simulink model "Model_samochodu"  (R2013a)
settings: Solver=ode113  StartTime=0.0  StopTime=1000  FixedStep=0.001  RelTol=1e-3
undefined symbols (not defined in the file): sigbuilder_block
settings Model: Creator=Damian  LastModifiedBy=Damian
settings SolverCC: ShapePreserveControl=EnableAll
settings DataIOCC: SignalLoggingSaveFormat=ModelDataLogs
settings OptimizationCC: BooleanDataType=off  InitFltsAndDblsToZero=on
settings HardwareCC: TargetHWDeviceType=32-bit Generic
settings GRTTargetCC: CombineOutputUpdateFcns=off  GRTInterface=on

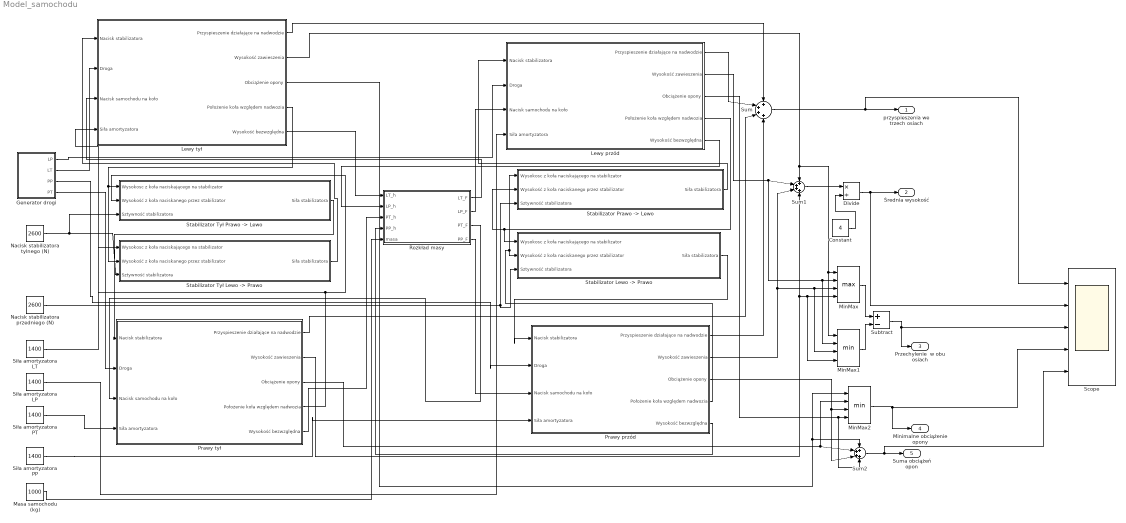
== system Model_samochodu ==
  Constant : Constant  Value=4
  Divide : Product  Inputs=*/
  Generator drogi : Subsystem
  Lewy przód : Subsystem
  Lewy tył : Subsystem
  Masa samochodu (kg) : Constant  Value=1000
  MinMax : MinMax  Function=max  Inputs=4
  MinMax1 : MinMax  Inputs=4
  MinMax2 : MinMax  Inputs=4
  Nacisk stabilizatora przedniego (N) : Constant  Value=2600
  Nacisk stabilizatora tylnego (N) : Constant  Value=2600
  Prawy przód : Subsystem
  Prawy tył : Subsystem
  Rozkład masy : Subsystem
  Scope : Scope  NumInputPorts=5
      settings: YMin=-5~-5~-5~-5~-5  YMax=5~5~5~5~5  SaveName=ScopeData6
  Siła amortyzatora LP : Constant  Value=1400
  Siła amortyzatora LT : Constant  Value=1400
  Siła amortyzatora PP : Constant  Value=1400
  Siła amortyzatora PT : Constant  Value=1400
  "Stabilizator Lewo -> Prawo" : Subsystem
  "Stabilizator Prawo -> Lewo" : Subsystem
  "Stabilizator Tył Lewo -> Prawo" : Subsystem
  "Stabilizator Tył Prawo -> Lewo" : Subsystem
  Subtract : Sum  Inputs=+-
  Sum : Sum  Inputs=++++
  Sum1 : Sum  Inputs=++++
  Sum2 : Sum  Inputs=++++
  przyspieszenia we trzech osiach : Outport
  "Średnia wysokość " : Outport  Port=2
  Przechylenie  w obu osiach : Outport  Port=3
  Minimalne obciążenie opony : Outport  Port=4
  "Suma obciążeń opon " : Outport  Port=5
  wires:
  Generator drogi/2(LT) -> Lewy tył/2(Droga)
  Generator drogi/1(LP) -> Lewy przód/2(Droga)
  Generator drogi/4(PT) -> Prawy tył/2(Droga)
  Generator drogi/3(PP) -> Prawy przód/2(Droga)
  Masa samochodu (kg)/1 -> Rozkład masy/5(masa)
  Rozkład masy/1(LT_F) -> Lewy tył/3(Nacisk samochodu na koło)
  Rozkład masy/2(LP_F) -> Lewy przód/3(Nacisk samochodu na koło)
  Rozkład masy/3(PT_F) -> Prawy tył/3(Nacisk samochodu na koło)
  Rozkład masy/4(PP_F) -> Prawy przód/3(Nacisk samochodu na koło)
  Lewy przód/4(Położenie koła względem nadwozia) -> "Stabilizator Prawo -> Lewo"/2(Wysokość z koła naciskanego przez stabilizator), "Stabilizator Lewo -> Prawo"/1(Wysokosc z koła naciskającego na stabilizator)
  Prawy przód/4(Położenie koła względem nadwozia) -> "Stabilizator Prawo -> Lewo"/1(Wysokosc z koła naciskającego na stabilizator), "Stabilizator Lewo -> Prawo"/2(Wysokość z koła naciskanego przez stabilizator)
  "Stabilizator Lewo -> Prawo"/1(Siła stabilizatora) -> Prawy przód/1(Nacisk stabilizatora)
  "Stabilizator Prawo -> Lewo"/1(Siła stabilizatora) -> Lewy przód/1(Nacisk stabilizatora)
  Lewy tył/4(Położenie koła względem nadwozia) -> "Stabilizator Tył Lewo -> Prawo"/2(Wysokość z koła naciskanego przez stabilizator), "Stabilizator Tył Prawo -> Lewo"/1(Wysokosc z koła naciskającego na stabilizator)
  Prawy tył/4(Położenie koła względem nadwozia) -> "Stabilizator Tył Prawo -> Lewo"/2(Wysokość z koła naciskanego przez stabilizator), "Stabilizator Tył Lewo -> Prawo"/1(Wysokosc z koła naciskającego na stabilizator)
  "Stabilizator Tył Prawo -> Lewo"/1(Siła stabilizatora) -> Prawy tył/1(Nacisk stabilizatora)
  "Stabilizator Tył Lewo -> Prawo"/1(Siła stabilizatora) -> Lewy tył/1(Nacisk stabilizatora)
  Nacisk stabilizatora tylnego (N)/1 -> "Stabilizator Tył Lewo -> Prawo"/3(Sztywność stabilizatora), "Stabilizator Tył Prawo -> Lewo"/3(Sztywność stabilizatora)
  Nacisk stabilizatora przedniego (N)/1 -> "Stabilizator Lewo -> Prawo"/3(Sztywność stabilizatora), "Stabilizator Prawo -> Lewo"/3(Sztywność stabilizatora)
  Siła amortyzatora LT/1 -> Lewy tył/4(Siła amortyzatora)
  Siła amortyzatora PT/1 -> Prawy tył/4(Siła amortyzatora)
  Siła amortyzatora LP/1 -> Lewy przód/4(Siła amortyzatora)
  Siła amortyzatora PP/1 -> Prawy przód/4(Siła amortyzatora)
  Lewy tył/5("Wysokość bezwzględna ") -> Rozkład masy/1(LT_h)
  Lewy przód/5("Wysokość bezwzględna ") -> Rozkład masy/2(LP_h)
  Prawy tył/5("Wysokość bezwzględna ") -> Rozkład masy/3(PT_h)
  Prawy przód/5("Wysokość bezwzględna ") -> Rozkład masy/4(PP_h)
  Lewy tył/1(Przyspieszenie działające na nadwodzie) -> Sum/1
  Lewy przód/1(Przyspieszenie działające na nadwodzie) -> Sum/2
  Prawy tył/1(Przyspieszenie działające na nadwodzie) -> Sum/3
  Prawy przód/1(Przyspieszenie działające na nadwodzie) -> Sum/4
  Sum/1 -> Scope/1, przyspieszenia we trzech osiach/1
  Lewy tył/2(Wysokość zawieszenia) -> MinMax/1, MinMax1/1, Sum1/1
  Lewy przód/2(Wysokość zawieszenia) -> MinMax1/2, MinMax/2, Sum1/2
  Prawy przód/2(Wysokość zawieszenia) -> MinMax1/3, MinMax/3, Sum1/3
  Prawy tył/2(Wysokość zawieszenia) -> MinMax1/4, MinMax/4, Sum1/4
  Sum1/1 -> Divide/1
  Constant/1 -> Divide/2
  Divide/1 -> "Średnia wysokość "/1, Scope/2
  MinMax/1 -> Subtract/1
  MinMax1/1 -> Subtract/2
  Subtract/1 -> Scope/3, Przechylenie  w obu osiach/1
  Lewy tył/3(Obciążenie opony) -> MinMax2/1, Sum2/1
  Prawy tył/3(Obciążenie opony) -> MinMax2/2, Sum2/2
  Prawy przód/3(Obciążenie opony) -> Sum2/3, MinMax2/3
  Lewy przód/3(Obciążenie opony) -> Sum2/4, MinMax2/4
  MinMax2/1 -> Scope/4, Minimalne obciążenie opony/1
  Sum2/1 -> Scope/5, "Suma obciążeń opon "/1

== system Model_samochodu/Generator drogi ==
  Signal Builder : Subsystem  Tag=STV Subsys  LoadFcn=sigbuilder_block('load');  StartFcn=sigbuilder_block('start');  StopFcn=sigbuilder_block('stop');  ClipboardFcn=sigbuilder_block('clipboard');  mask(Sigbuilder block){}
      mask help: Create and generate interchangeable groups of signals whose waveforms are piecewise linear.
      mask init:
      | if ~strcmp(get_param(bdroot(gcbh),'SimulationStatus'),'stopped') tuvar = sigbuilder_block('maskInit'); end
      settings: CopyFcn=sigbuilder_block('copy');  DeleteFcn=sigbuilder_block('delete');  ModelCloseFcn=sigbuilder_block('modelClose');  PreSaveFcn=sigbuilder_block('preSave');  PauseFcn=sigbuilder_block('pause')  ContinueFcn=sigbuilder_block('continue')  NameChangeFcn=sigbuilder_block('namechange');  OpenFcn=sigbuilder_block('open',[108 122.25 550.5 390 ]);  CloseFcn=sigbuilder_block('close');
      mask Display: plot(0,0,100,100,[10,10,40,40,10],[80,20,20,80,80],[40,10],[50,50], [40,27,10],[65,72,56],[40,25,25,10],[28,28,43,43]);
  Signal Builder1 : Subsystem  Tag=STV Subsys  LoadFcn=sigbuilder_block('load');  StartFcn=sigbuilder_block('start');  StopFcn=sigbuilder_block('stop');  ClipboardFcn=sigbuilder_block('clipboard');  mask(Sigbuilder block){}
      mask help: Simulink:masks:SigbuilderBlock_MD
      mask init:
      | if ~strcmp(get_param(bdroot(gcbh),'SimulationStatus'),'stopped') tuvar = sigbuilder_block('maskInit'); end
      settings: CopyFcn=sigbuilder_block('copy');  DeleteFcn=sigbuilder_block('delete');  ModelCloseFcn=sigbuilder_block('modelClose');  PreSaveFcn=sigbuilder_block('preSave');  PauseFcn=sigbuilder_block('pause');  ContinueFcn=sigbuilder_block('continue');  NameChangeFcn=sigbuilder_block('namechange');  OpenFcn=sigbuilder_block('open',[0 30 1258.5 678.75 ]);  CloseFcn=sigbuilder_block('close');
      mask Display: plot(0, 0, 100, 100,[2, 2, 32, 32, 2], [68, 8, 8, 68, 68],[32, 2], [38, 38], [32, 19, 2],[53, 60, 44], [32, 17, 17, 2],[16, 16, 31, 31]);txt = getActiveGroup(gcbh);text(2, 100, txt,'verticalAlignment', 'top');
  Transport Delay1 : TransportDelay  DelayTime=0.27  BufferSize=102400
  Transport Delay2 : TransportDelay  DelayTime=0.27  BufferSize=102400
  LP : Outport
  LT : Outport  Port=2
  PP : Outport  Port=3
  PT : Outport  Port=4
  wires:
  Signal Builder1/1(Lewe koło) -> Transport Delay1/1, LP/1
  Transport Delay1/1 -> LT/1
  Transport Delay2/1 -> PT/1
  Signal Builder1/2(Prawe koło) -> Transport Delay2/1, PP/1

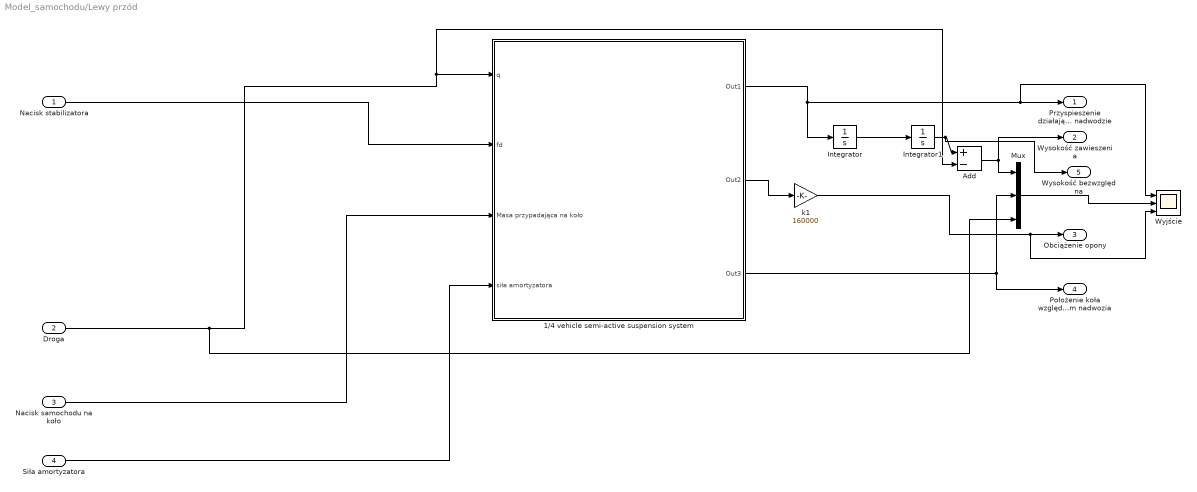
== system Model_samochodu/Lewy przód ==
  Nacisk stabilizatora : Inport
  Droga : Inport  Port=2
  Nacisk samochodu na koło : Inport  Port=3
  Siła amortyzatora : Inport  Port=4
  1/4 vehicle semi-active suspension system : Subsystem
      mask Display: image(imread('Semi_acitve model2DOF.jpg'));
  Add : Sum  Inputs=+-
  Integrator : Integrator
  Integrator1 : Integrator
  Mux : Mux  Inputs=3
  Wyjście : Scope  NumInputPorts=3
      settings: YMin=-40~-0.4~-20000  YMax=40~0.4~20000  SaveName=ScopeData3
  k1 : Gain  Gain=160000  SaturateOnIntegerOverflow=on  OutDataTypeStr=Inherit: Same as input  ParamDataTypeStr=Inherit: Same as input
  Przyspieszenie działające na nadwodzie : Outport
  Wysokość zawieszenia : Outport  Port=2
  Obciążenie opony : Outport  Port=3
  Położenie koła względem nadwozia : Outport  Port=4
  "Wysokość bezwzględna " : Outport  Port=5
  wires:
  1/4 vehicle semi-active suspension system/1(Out1) -> Integrator/1, Wyjście/1, Przyspieszenie działające na nadwodzie/1
  1/4 vehicle semi-active suspension system/3(Out3) -> Mux/2, Położenie koła względem nadwozia/1
  1/4 vehicle semi-active suspension system/2(Out2) -> k1/1
  k1/1 -> Wyjście/3, Obciążenie opony/1
  Integrator/1 -> Integrator1/1
  Mux/1 -> Wyjście/2
  Droga/1 -> Mux/3, 1/4 vehicle semi-active suspension system/1(q), Add/2
  Nacisk samochodu na koło/1 -> 1/4 vehicle semi-active suspension system/3(Masa przypadająca na koło)
  Nacisk stabilizatora/1 -> 1/4 vehicle semi-active suspension system/2(fd)
  Integrator1/1 -> "Wysokość bezwzględna "/1, Add/1
  Add/1 -> Mux/1, Wysokość zawieszenia/1
  Siła amortyzatora/1 -> 1/4 vehicle semi-active suspension system/4(siła amortyzatora)

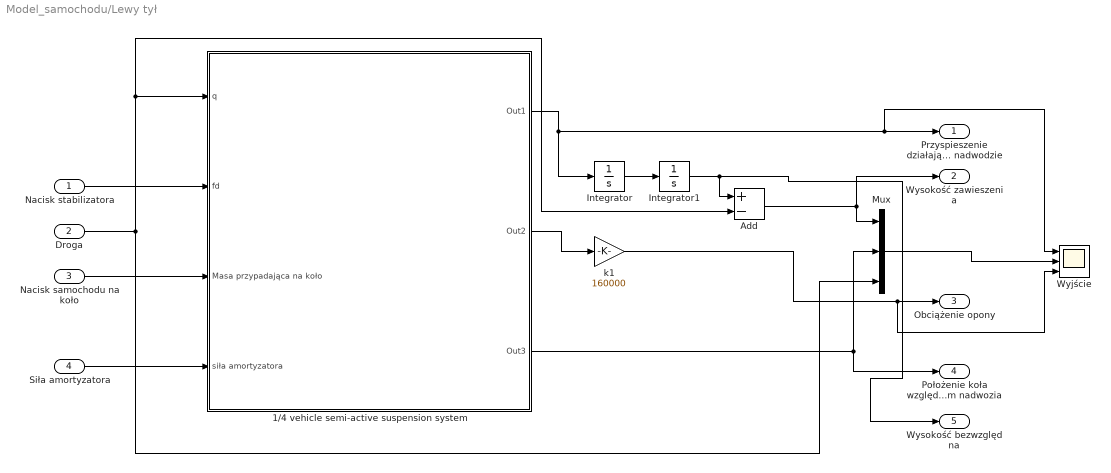
== system Model_samochodu/Lewy tył ==
  Nacisk stabilizatora : Inport
  Droga : Inport  Port=2
  Nacisk samochodu na koło : Inport  Port=3
  Siła amortyzatora : Inport  Port=4
  1/4 vehicle semi-active suspension system : Subsystem
      mask Display: image(imread('Semi_acitve model2DOF.jpg'));
  Add : Sum  Inputs=+-
  Integrator : Integrator
  Integrator1 : Integrator
  Mux : Mux  Inputs=3
  Wyjście : Scope  NumInputPorts=3
      settings: YMin=-40~-0.4~-20000  YMax=40~0.4~20000
  k1 : Gain  Gain=160000  SaturateOnIntegerOverflow=on  OutDataTypeStr=Inherit: Same as input  ParamDataTypeStr=Inherit: Same as input
  Przyspieszenie działające na nadwodzie : Outport
  Wysokość zawieszenia : Outport  Port=2
  Obciążenie opony : Outport  Port=3
  Położenie koła względem nadwozia : Outport  Port=4
  "Wysokość bezwzględna " : Outport  Port=5
  wires:
  1/4 vehicle semi-active suspension system/1(Out1) -> Wyjście/1, Przyspieszenie działające na nadwodzie/1, Integrator/1
  1/4 vehicle semi-active suspension system/3(Out3) -> Mux/2, Położenie koła względem nadwozia/1
  1/4 vehicle semi-active suspension system/2(Out2) -> k1/1
  k1/1 -> Wyjście/3, Obciążenie opony/1
  Integrator/1 -> Integrator1/1
  Mux/1 -> Wyjście/2
  Droga/1 -> 1/4 vehicle semi-active suspension system/1(q), Add/2, Mux/3
  Nacisk samochodu na koło/1 -> 1/4 vehicle semi-active suspension system/3(Masa przypadająca na koło)
  Nacisk stabilizatora/1 -> 1/4 vehicle semi-active suspension system/2(fd)
  Integrator1/1 -> "Wysokość bezwzględna "/1, Add/1
  Add/1 -> Mux/1, Wysokość zawieszenia/1
  Siła amortyzatora/1 -> 1/4 vehicle semi-active suspension system/4(siła amortyzatora)

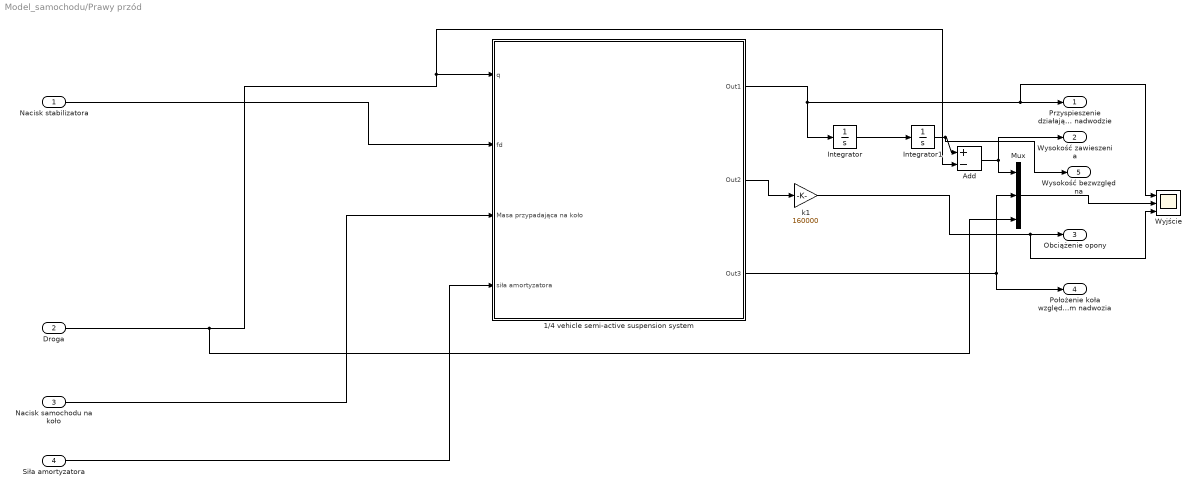
== system Model_samochodu/Prawy przód ==
  Nacisk stabilizatora : Inport
  Droga : Inport  Port=2
  Nacisk samochodu na koło : Inport  Port=3
  Siła amortyzatora : Inport  Port=4
  1/4 vehicle semi-active suspension system : Subsystem
      mask Display: image(imread('Semi_acitve model2DOF.jpg'));
  Add : Sum  Inputs=+-
  Integrator : Integrator
  Integrator1 : Integrator
  Mux : Mux  Inputs=3
  Wyjście : Scope  NumInputPorts=3
      settings: YMin=-40~-0.4~-20000  YMax=40~0.4~20000  SaveName=ScopeData5
  k1 : Gain  Gain=160000  SaturateOnIntegerOverflow=on  OutDataTypeStr=Inherit: Same as input  ParamDataTypeStr=Inherit: Same as input
  Przyspieszenie działające na nadwodzie : Outport
  Wysokość zawieszenia : Outport  Port=2
  Obciążenie opony : Outport  Port=3
  Położenie koła względem nadwozia : Outport  Port=4
  "Wysokość bezwzględna " : Outport  Port=5
  wires:
  1/4 vehicle semi-active suspension system/1(Out1) -> Integrator/1, Wyjście/1, Przyspieszenie działające na nadwodzie/1
  1/4 vehicle semi-active suspension system/3(Out3) -> Mux/2, Położenie koła względem nadwozia/1
  1/4 vehicle semi-active suspension system/2(Out2) -> k1/1
  k1/1 -> Wyjście/3, Obciążenie opony/1
  Integrator/1 -> Integrator1/1
  Mux/1 -> Wyjście/2
  Droga/1 -> Mux/3, 1/4 vehicle semi-active suspension system/1(q), Add/2
  Nacisk samochodu na koło/1 -> 1/4 vehicle semi-active suspension system/3(Masa przypadająca na koło)
  Nacisk stabilizatora/1 -> 1/4 vehicle semi-active suspension system/2(fd)
  Integrator1/1 -> "Wysokość bezwzględna "/1, Add/1
  Add/1 -> Mux/1, Wysokość zawieszenia/1
  Siła amortyzatora/1 -> 1/4 vehicle semi-active suspension system/4(siła amortyzatora)

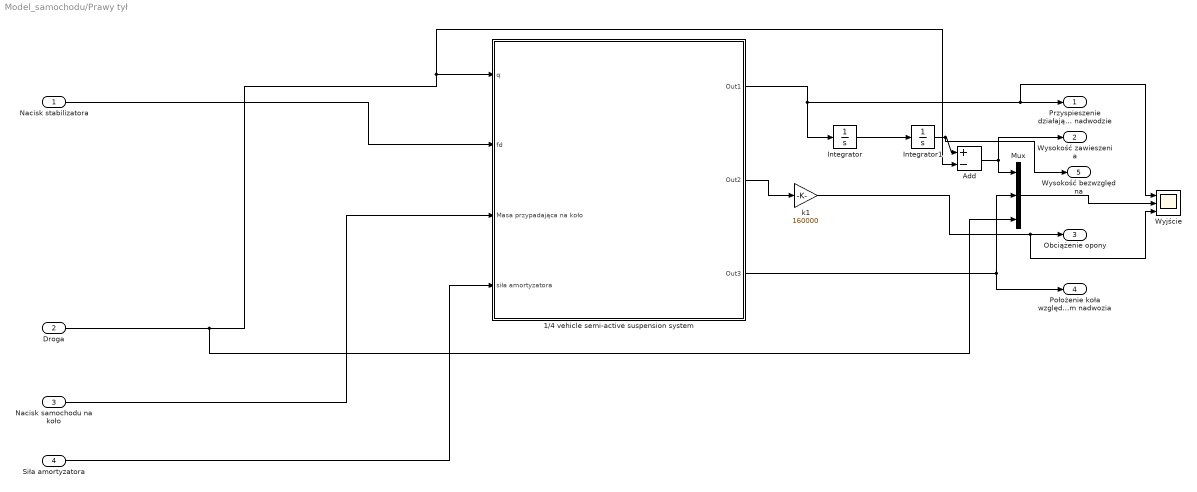
== system Model_samochodu/Prawy tył ==
  Nacisk stabilizatora : Inport
  Droga : Inport  Port=2
  Nacisk samochodu na koło : Inport  Port=3
  Siła amortyzatora : Inport  Port=4
  1/4 vehicle semi-active suspension system : Subsystem
      mask Display: image(imread('Semi_acitve model2DOF.jpg'));
  Add : Sum  Inputs=+-
  Integrator : Integrator
  Integrator1 : Integrator
  Mux : Mux  Inputs=3
  Wyjście : Scope  NumInputPorts=3
      settings: YMin=-40~-0.4~-20000  YMax=40~0.4~20000  SaveName=ScopeData2
  k1 : Gain  Gain=160000  SaturateOnIntegerOverflow=on  OutDataTypeStr=Inherit: Same as input  ParamDataTypeStr=Inherit: Same as input
  Przyspieszenie działające na nadwodzie : Outport
  Wysokość zawieszenia : Outport  Port=2
  Obciążenie opony : Outport  Port=3
  Położenie koła względem nadwozia : Outport  Port=4
  "Wysokość bezwzględna " : Outport  Port=5
  wires:
  1/4 vehicle semi-active suspension system/1(Out1) -> Integrator/1, Wyjście/1, Przyspieszenie działające na nadwodzie/1
  1/4 vehicle semi-active suspension system/3(Out3) -> Mux/2, Położenie koła względem nadwozia/1
  1/4 vehicle semi-active suspension system/2(Out2) -> k1/1
  k1/1 -> Wyjście/3, Obciążenie opony/1
  Integrator/1 -> Integrator1/1
  Mux/1 -> Wyjście/2
  Droga/1 -> Mux/3, 1/4 vehicle semi-active suspension system/1(q), Add/2
  Nacisk samochodu na koło/1 -> 1/4 vehicle semi-active suspension system/3(Masa przypadająca na koło)
  Nacisk stabilizatora/1 -> 1/4 vehicle semi-active suspension system/2(fd)
  Integrator1/1 -> "Wysokość bezwzględna "/1, Add/1
  Add/1 -> Mux/1, Wysokość zawieszenia/1
  Siła amortyzatora/1 -> 1/4 vehicle semi-active suspension system/4(siła amortyzatora)

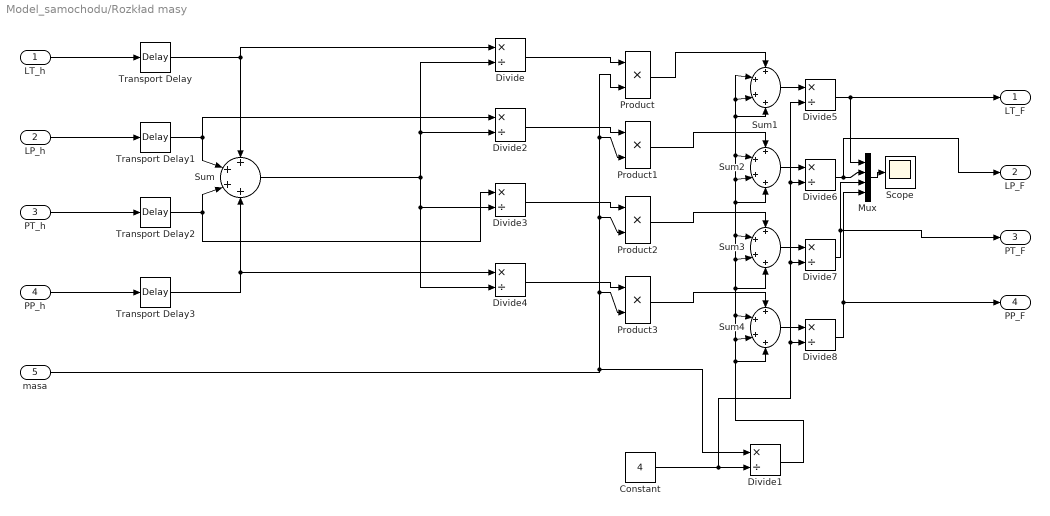
== system Model_samochodu/Rozkład masy ==
  LT_h : Inport
  LP_h : Inport  Port=2
  PT_h : Inport  Port=3
  PP_h : Inport  Port=4
  masa : Inport  Port=5
  Constant : Constant  Value=4
  Divide{,1..8} (9 alike) : Product  Inputs=*/
  Mux : Mux
  Product{,1..3} (4 alike) : Product
  Scope : Scope
      settings: TimeRange=1000  YMin=170  YMax=330
  Sum{,1..4} (5 alike) : Sum  Inputs=++++
  Transport Delay{,1..3} (4 alike) : TransportDelay  DelayTime=0.001  InitialOutput=1
  LT_F : Outport
  LP_F : Outport  Port=2
  PT_F : Outport  Port=3
  PP_F : Outport  Port=4
  wires:
  Sum/1 -> Divide4/2, Divide3/2, Divide2/2, Divide/2
  Divide/1 -> Product/1
  Divide2/1 -> Product1/1
  Divide3/1 -> Product2/1
  Divide4/1 -> Product3/1
  masa/1 -> Divide1/1, Product3/2, Product2/2, Product1/2, Product/2
  Mux/1 -> Scope/1
  Constant/1 -> Divide5/2, Divide6/2, Divide7/2, Divide8/2, Divide1/2
  Transport Delay/1 -> Sum/1, Divide/1
  Transport Delay1/1 -> Divide2/1, Sum/2
  Transport Delay2/1 -> Sum/3, Divide3/1
  Transport Delay3/1 -> Divide4/1, Sum/4
  LT_h/1 -> Transport Delay/1
  LP_h/1 -> Transport Delay1/1
  PT_h/1 -> Transport Delay2/1
  PP_h/1 -> Transport Delay3/1
  Product/1 -> Sum1/1
  Product1/1 -> Sum2/1
  Divide1/1 -> Sum4/4, Sum4/2, Sum3/4, Sum3/2, Sum2/4, Sum2/2, Sum1/4, Sum1/3, Sum1/2, Sum2/3, Sum3/3, Sum4/3
  Product2/1 -> Sum3/1
  Product3/1 -> Sum4/1
  Sum1/1 -> Divide5/1
  Sum2/1 -> Divide6/1
  Sum3/1 -> Divide7/1
  Sum4/1 -> Divide8/1
  Divide5/1 -> LT_F/1, Mux/1
  Divide8/1 -> PP_F/1, Mux/4
  Divide6/1 -> LP_F/1, Mux/2
  Divide7/1 -> PT_F/1, Mux/3

== system Model_samochodu/Stabilizator Lewo -> Prawo ==
  Wysokosc z koła naciskającego na stabilizator : Inport
  Wysokość z koła naciskanego przez stabilizator : Inport  Port=2
  Sztywność stabilizatora : Inport  Port=3
  Divide : Product  Inputs=**
  Gain : Gain  Gain=-1
  Subtract : Sum  Inputs=+-
  Siła stabilizatora : Outport
  wires:
  Wysokosc z koła naciskającego na stabilizator/1 -> Subtract/1
  Wysokość z koła naciskanego przez stabilizator/1 -> Subtract/2
  Subtract/1 -> Divide/1
  Sztywność stabilizatora/1 -> Divide/2
  Divide/1 -> Gain/1
  Gain/1 -> Siła stabilizatora/1

== system Model_samochodu/Stabilizator Prawo -> Lewo ==
  Wysokosc z koła naciskającego na stabilizator : Inport
  Wysokość z koła naciskanego przez stabilizator : Inport  Port=2
  Sztywność stabilizatora : Inport  Port=3
  Divide : Product  Inputs=**
  Gain : Gain  Gain=-1
  Subtract : Sum  Inputs=+-
  Siła stabilizatora : Outport
  wires:
  Wysokosc z koła naciskającego na stabilizator/1 -> Subtract/1
  Wysokość z koła naciskanego przez stabilizator/1 -> Subtract/2
  Subtract/1 -> Divide/1
  Sztywność stabilizatora/1 -> Divide/2
  Divide/1 -> Gain/1
  Gain/1 -> Siła stabilizatora/1

== system Model_samochodu/Stabilizator Tył Lewo -> Prawo ==
  Wysokosc z koła naciskającego na stabilizator : Inport
  Wysokość z koła naciskanego przez stabilizator : Inport  Port=2
  Sztywność stabilizatora : Inport  Port=3
  Divide : Product  Inputs=**
  Gain : Gain  Gain=-1
  Subtract : Sum  Inputs=+-
  Siła stabilizatora : Outport
  wires:
  Wysokosc z koła naciskającego na stabilizator/1 -> Subtract/1
  Wysokość z koła naciskanego przez stabilizator/1 -> Subtract/2
  Subtract/1 -> Divide/1
  Sztywność stabilizatora/1 -> Divide/2
  Divide/1 -> Gain/1
  Gain/1 -> Siła stabilizatora/1

== system Model_samochodu/Stabilizator Tył Prawo -> Lewo ==
  Wysokosc z koła naciskającego na stabilizator : Inport
  Wysokość z koła naciskanego przez stabilizator : Inport  Port=2
  Sztywność stabilizatora : Inport  Port=3
  Divide : Product  Inputs=**
  Gain : Gain  Gain=-1
  Subtract : Sum  Inputs=+-
  Siła stabilizatora : Outport
  wires:
  Wysokosc z koła naciskającego na stabilizator/1 -> Subtract/1
  Wysokość z koła naciskanego przez stabilizator/1 -> Subtract/2
  Subtract/1 -> Divide/1
  Sztywność stabilizatora/1 -> Divide/2
  Divide/1 -> Gain/1
  Gain/1 -> Siła stabilizatora/1

== system Model_samochodu/Generator drogi/Signal Builder ==
  Demux : Demux  Tag=STV Demux  Outputs=2
  FromWs : FromWorkspace  Tag=STV FromWs  VariableName=tuvar  SampleTime=0
      SigBuilderData=|
      | common.afterFinalStr = 'Extrapolate'
      | common.sampleTime = 0
      | dataSet.timeRange = [0 100]
      | dataSet.name = 'Arkusz1'
      | sbobj.Name = 'Signal Builder'
      | sbobj.Groups.Name = 'Arkusz1'
      | sbobj.Groups.Signals(1).Name = 'Imported_Signal 1'
      | sbobj.Groups.Signals(1).XData = [0 44.5 45 48 48 100]
      | sbobj.Groups.Signals(1).YData = [0 0 0.1 0.1 -0.001 0]
      | sbobj.Groups.Signals(2).Name = 'Imported_Signal 2'
      | sbobj.Groups.Signals(2).XData = [0 10 15 20 30 31 32 33 34 35 36 37 38 39 50 51 52 53 54 55 56 57 58 59 60 70 75 80 85 90 95 100]
      | sbobj.Groups.Signals(2).YData = [0 0.1 0.1 0 0.01 0.014 0.02 0.032 0.06 0.072 0.078 0.084 0.09 0.1 0.1 0.096 0.09 0.082 0.07 0.038 0.016 0.01 0.01 0.016 0.006 -0.1 -0.05 -0.05 0.02 0.03 0.02 0]
      | sbobj.Groups.TimeRange = [0 100]
  Imported_Signal 1 : Outport
  Imported_Signal 2 : Outport  Tag=STV Outport  Port=2
  wires:
  FromWs/1 -> Demux/1
  Demux/1 -> Imported_Signal 1/1
  Demux/2 -> Imported_Signal 2/1

== system Model_samochodu/Generator drogi/Signal Builder1 ==
  Demux : Demux  Tag=STV Demux  Outputs=2
  FromWs : FromWorkspace  Tag=STV FromWs  VariableName=tuvar  SampleTime=0
      SigBuilderData=|
      | common.afterFinalStr = 'Extrapolate'
      | common.sampleTime = 0
      | dataSet.timeRange = [0 1000]
      | dataSet.name = 'Group 1'
      | sbobj.Groups.Name = 'Group 1'
      | sbobj.Groups.Signals(1).Name = 'Lewe koło'
      | sbobj.Groups.Signals(1).XData = [0 20 20.5 21 22 40 40 41.5 42 60 60 61.5 61.5 75 75.5 76 76 77 77 78 78.5 79 79.5 80 80 81 81.5 82 82.5 83 83.5 84 84.5 85 85.5 86.5 87 88 89.5 90.5 91 91.5 92 93 93.5 94.5 95 95.5 96.5 97 97.5 98 110 110 111 111 112 112 113 113 114 114 115 115 130 131 133 135.5 137.5 138.5 140 160 161 164 167 170 172 190 190.5 191 191 192 192.5 193 206 207 208 208.5 209.5 210 211 212 213 227 228 229 230 230.5 231 231.5 232 232.5 233 233 233.5 235.5 236 237.5 238.5 239 240 241 247.5 248.5 249.5 250 251 252 252.5 253 269.5 271 273 275 277 278 280.5 283 285.5 288.5 291 294.5 297 300 303 308 312 313.5 315 317 318 319.5 321 328 331.5 334.5 338 344 344 358.5 359.5 361.5 363 364 366 367.5 369.5 371.5 374 377 379 382 384 385 400.5 400.5 403.5 403.5 415 415 417.5 417.5 432 432 435 436.5 439 440 442 446 449 480 481 483 484.5 487 489 491 493 495.5 498 500 501.5 504 505.5 506.5 508.5 509 510 524 564 571 628 660.5 660.5 664 664 668 668 671.5 671.5 676 676 679 679 682.5 682.5 686 686 689.5 689.5 692.5 692.5 697 697 701 701 706 706 711 711 715.5 715.5 720.5 720.5 751 753 756.5 760 763 767 771 774.5 778 782 787 791 796 799 800.3 800.3 800.5 800.5 800.75 800.75 801.05 801.05 801.2 801.2 801.35 801.35 801.5 801.5 801.6 801.6 801.75 801.75 801.95 801.95 802.2 802.2 802.4 802.4 802.7 802.7 802.95 802.95 803.2 803.2 803.5 803.5 803.7 803.7 803.85 803.85 804 804 804.2 804.2 804.4 804.4 804.65 804.65 804.85 804.85 805.1 805.1 805.36 805.36 805.58 805.58 805.72 805.72 805.92 805.92 806.06 806.06 806.22 806.22 806.38 806.38 806.56 806.56 806.78 806.78 806.94 806.94 807.08 807.08 807.24 807.24 807.44 807.44 807.6 807.6 807.78 807.78 807.98 807.98 810 814.5 815.8 820 825 829 834 841 843.2 846.5 851.5 856 862 867.8 867.8 872.8 872.8 877.2 879.6 887.4 893 899 904.6 910.4 917 923.4 930.4 936.2 942.6 948 954.8 959.4 965 971.6 977 984.6 989.6 994.2 1000]
      | sbobj.Groups.Signals(1).YData = [0.001 0.001 0.101 0.101 0.001 0.001 -0.1 -0.1 0 0 0.101 0.101 ... (368 elements, 1x368)]
      | sbobj.Groups.Signals(2).Name = 'Prawe koło'
      | sbobj.Groups.Signals(2).XData = [0 19.5 20 20.5 21 39.5 40 41 41.5 59.5 60 61 61.5 74.5 75 75.5 76.5 77.5 78.5 79.5 80.5 82 83 84 85 85 86 86.5 87.5 88.5 89.5 90 90.5 91.5 92.5 93.5 93.5 94.5 109.5 109.5 110.5 110.5 111 111 112 112 113.5 113.5 114.5 114.5 129.5 130.5 132.5 135 136.5 138.5 139.5 159.5 160.5 163.5 166.5 169.5 171 189.5 190 190.5 191 191.5 192 193 193.5 226.5 226.5 227.5 227.5 229.5 229.5 230.5 230.5 231 231 240 240 241.5 241.5 246.5 250 252 264.5 266.5 266.5 274 278.5 288.5 295.5 311.5 324 342.5 342.5 358 358 359 359 359.5 359.5 360.5 360.5 361.5 361.5 362 362 363 363 364 364 365 365 366 366 367.5 367.5 368 368 368.5 368.5 369.5 369.5 370.5 370.5 372 372 373 373 375 375 408.5 408.5 411 411 423 423 432 432 435 438 440.5 444 446.5 449 452.5 479.5 481 482.5 485.5 487.5 489.5 491 494.5 497 499.5 502 505.5 507 508.5 509.5 519.5 519.5 525 525 529.5 529.5 533 533 538 538 542.5 542.5 545.5 545.5 549.5 549.5 554.5 554.5 559 559 564 564 568.5 568.5 574.5 574.5 579.5 579.5 584 584 589.5 589.5 596 596 601 601 609 609 613.5 613.5 617.5 617.5 621.5 621.5 626 626 659.5 663.5 667.5 671.5 675.5 680 684.5 689.5 695 699.5 705 710 715 720 748 752.5 757 762 762 766 766 769 773 777 780.5 786.5 791.5 796.5 800 800.18 800.18 800.32 800.32 800.42 800.42 800.52 800.52 800.66 800.66 800.82 800.82 800.92 800.92 801.02 801.02 801.12 801.12 801.24 801.24 801.34 801.34 801.44 801.44 801.58 801.58 801.76 801.76 801.84 801.84 801.96 801.96 802.04 802.04 802.18 802.18 802.34 802.34 802.48 802.48 802.64 802.64 802.84 803.06 803.24 803.24 803.41 803.41 803.58 804 804 805.15 805.15 805.27 805.27 805.85 805.85 806.03 806.03 806.3 807 807 807.52 807.74 807.74 808.02 808.02 808.28 811.5 816.5 821 826 830.5 834 839.5 845 850 855 859 864.5 864.5 870 870 874.5 876.5 879.5 880.8 882.6 884.6 888.4 891.8 894 898.4 900.8 902.8 906.2 911 915 923.5 923.5 931 931 935.5 935.5 939 939 941 941 944 946.5 949.5 950.5 953.5 957 960 961.5 964 967 970 976 981 988 994 1000]
      | sbobj.Groups.Signals(2).YData = [-0.001 -0.001 0.099 0.099 -0.001 -0.001 -0.101 -0.1 -0.002 -0.001 -0.1 -0.099 ... (364 elements, 1x364)]
      | sbobj.Groups.TimeRange = [0 1000]
  Lewe koło : Outport  Tag=STV Outport
  Prawe koło : Outport  Tag=STV Outport  Port=2
  wires:
  Demux/1 -> Lewe koło/1
  FromWs/1 -> Demux/1
  Demux/2 -> Prawe koło/1

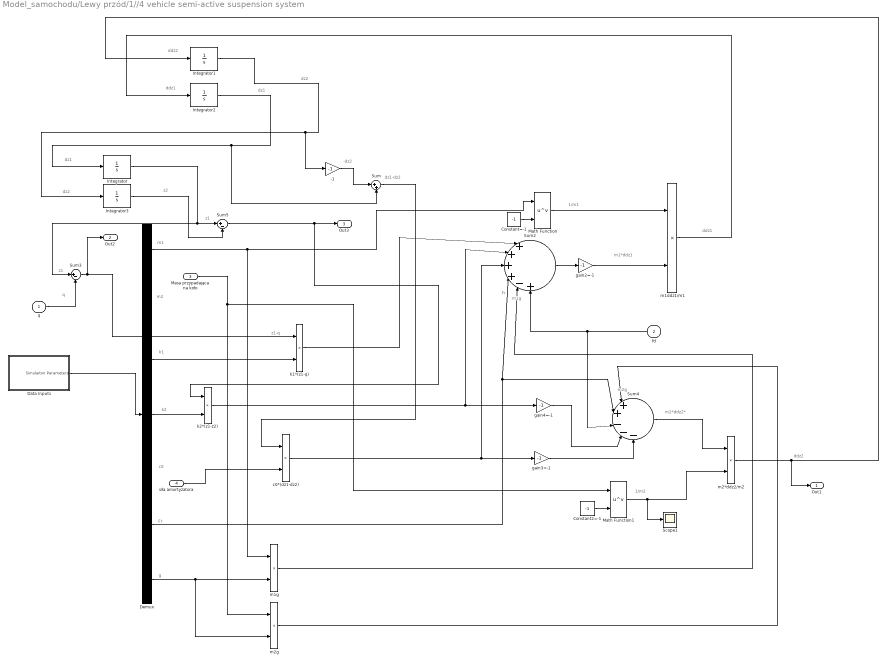
== system Model_samochodu/Lewy przód/1//4 vehicle semi-active suspension system ==
  note: m1
  note: k1
  note: m2
  note: k2
  note: c0
  note: z1
  note: dz1
  note: Fr
  note: g
  note: dz2
  note: -dz2
  note: dz1-dz2
  note: dz1
  note: dz2
  note: ddz2
  note: q
  note: z1
  note: z1-q
  note: Fr
  note: m1g
  note: m1*ddz1
  note: 1/m1
  note: ddz1
  note: m2g
  note: m2*ddz2*
  note: 1/m2
  note: ddz2
  note: z2
  note: ddz1
  q : Inport
  fd : Inport  Port=2
  Masa przypadająca na koło : Inport  Port=3
  siła amortyzatora : Inport  Port=4
  -1 : Gain  Gain=-1  SaturateOnIntegerOverflow=on  OutDataTypeStr=Inherit: Same as input  ParamDataTypeStr=Inherit: Same as input
  Constant2=-1 : Constant  Value=-1
  Constant=-1 : Constant  Value=-1
  Data Inputs : Subsystem
  Demux : Demux  Outputs=7
  Integrator{,1..3} (4 alike) : Integrator
  Math Function : Math  Operator=pow  SaturateOnIntegerOverflow=on
  Math Function1 : Math  Operator=pow  SaturateOnIntegerOverflow=on
  Scope1 : Scope
      settings: SaveName=ScopeData4
  Sum : Sum  Inputs=|++  SaturateOnIntegerOverflow=on  InputSameDT=on  OutDataTypeStr=Inherit: Same as first input
  Sum2 : Sum  Inputs=|++++-+  SaturateOnIntegerOverflow=on  InputSameDT=on  OutDataTypeStr=Inherit: Same as first input
  Sum3 : Sum  Inputs=|+-  SaturateOnIntegerOverflow=on  InputSameDT=on  OutDataTypeStr=Inherit: Same as first input
  Sum4 : Sum  Inputs=|++---  SaturateOnIntegerOverflow=on  InputSameDT=on  OutDataTypeStr=Inherit: Same as first input
  Sum5 : Sum  Inputs=|+-  SaturateOnIntegerOverflow=on  InputSameDT=on  OutDataTypeStr=Inherit: Same as first input
  c0*(dz1-dz2) : Product  SaturateOnIntegerOverflow=on  RndMeth=Zero  InputSameDT=on  OutDataTypeStr=Inherit: Same as first input
  gain2=-1 : Gain  Gain=-1  SaturateOnIntegerOverflow=on  OutDataTypeStr=Inherit: Same as input  ParamDataTypeStr=Inherit: Same as input
  gain3=-1 : Gain  Gain=-1  SaturateOnIntegerOverflow=on  OutDataTypeStr=Inherit: Same as input  ParamDataTypeStr=Inherit: Same as input
  gain4=-1 : Gain  Gain=-1  SaturateOnIntegerOverflow=on  OutDataTypeStr=Inherit: Same as input  ParamDataTypeStr=Inherit: Same as input
  k1*(z1-q) : Product  SaturateOnIntegerOverflow=on  RndMeth=Zero  InputSameDT=on  OutDataTypeStr=Inherit: Same as first input
  k2*(z1-z2) : Product  SaturateOnIntegerOverflow=on  RndMeth=Zero  InputSameDT=on  OutDataTypeStr=Inherit: Same as first input
  m1ddz1/m1 : Product  SaturateOnIntegerOverflow=on  RndMeth=Zero  InputSameDT=on  OutDataTypeStr=Inherit: Same as first input
  m1g : Product  SaturateOnIntegerOverflow=on  RndMeth=Zero  InputSameDT=on  OutDataTypeStr=Inherit: Same as first input
  m2*ddz2/m2 : Product  SaturateOnIntegerOverflow=on  RndMeth=Zero  InputSameDT=on  OutDataTypeStr=Inherit: Same as first input
  m2g : Product  SaturateOnIntegerOverflow=on  RndMeth=Zero  InputSameDT=on  OutDataTypeStr=Inherit: Same as first input
  Out1 : Outport
  Out2 : Outport  Port=2
  Out3 : Outport  Port=3
  wires:
  Data Inputs/1("Simulaiton Parameters ") -> Demux/1
  Demux/1 -> m1g/1, Math Function/1
  Integrator2/1 -> Sum/2, Integrator/1
  Integrator/1 -> Sum5/1, Sum3/1
  siła amortyzatora/1 -> c0*(dz1-dz2)/2
  -1/1 -> Sum/1
  Sum/1 -> c0*(dz1-dz2)/1
  Integrator1/1 -> -1/1, Integrator3/1
  Demux/4 -> k2*(z1-z2)/2
  Demux/3 -> k1*(z1-q)/2
  Sum3/1 -> k1*(z1-q)/1, Out2/1
  Sum2/1 -> gain2=-1/1
  gain2=-1/1 -> m1ddz1/m1/2
  k1*(z1-q)/1 -> Sum2/1
  k2*(z1-z2)/1 -> Sum2/2, gain4=-1/1
  c0*(dz1-dz2)/1 -> Sum2/3, gain3=-1/1
  fd/1 -> Sum2/6, Sum4/3
  Constant=-1/1 -> Math Function/2
  Math Function/1 -> m1ddz1/m1/1
  m1ddz1/m1/1 -> Integrator2/1
  Demux/6 -> Sum2/4, Sum4/2
  gain3=-1/1 -> Sum4/5
  gain4=-1/1 -> Sum4/4
  Sum4/1 -> m2*ddz2/m2/1
  Demux/7 -> m1g/2, m2g/2
  Masa przypadająca na koło/1 -> m2g/1, Math Function1/1
  m1g/1 -> Sum2/5
  m2g/1 -> Sum4/1
  Constant2=-1/1 -> Math Function1/2
  Math Function1/1 -> m2*ddz2/m2/2, Scope1/1
  m2*ddz2/m2/1 -> Integrator1/1, Out1/1
  Integrator3/1 -> Sum5/2
  Sum5/1 -> k2*(z1-z2)/1, Out3/1
  q/1 -> Sum3/2

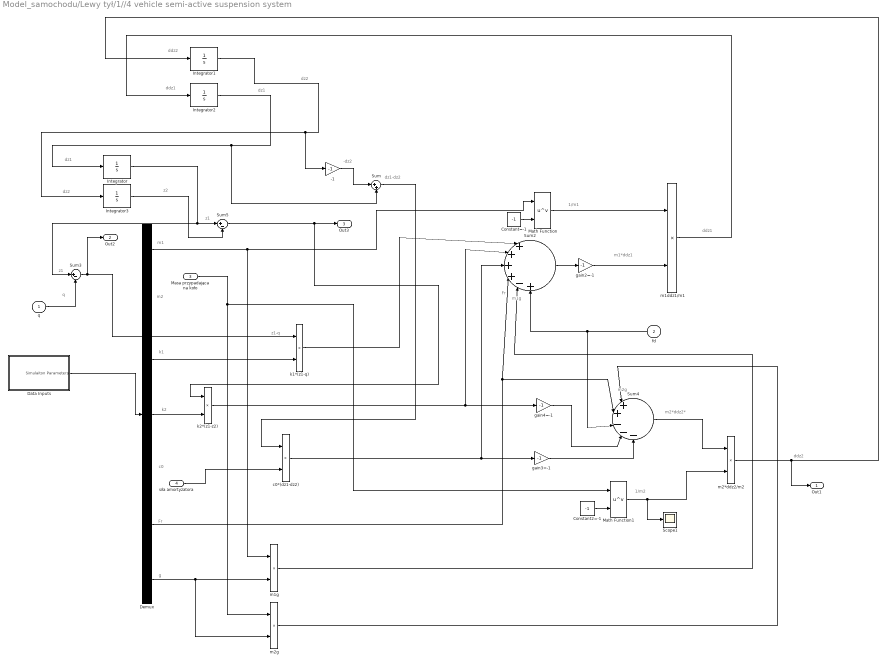
== system Model_samochodu/Lewy tył/1//4 vehicle semi-active suspension system ==
  note: m1
  note: k1
  note: m2
  note: k2
  note: c0
  note: z1
  note: dz1
  note: Fr
  note: g
  note: dz2
  note: -dz2
  note: dz1-dz2
  note: dz1
  note: dz2
  note: ddz2
  note: q
  note: z1
  note: z1-q
  note: Fr
  note: m1g
  note: m1*ddz1
  note: 1/m1
  note: ddz1
  note: m2g
  note: m2*ddz2*
  note: 1/m2
  note: ddz2
  note: z2
  note: ddz1
  q : Inport
  fd : Inport  Port=2
  Masa przypadająca na koło : Inport  Port=3
  siła amortyzatora : Inport  Port=4
  -1 : Gain  Gain=-1  SaturateOnIntegerOverflow=on  OutDataTypeStr=Inherit: Same as input  ParamDataTypeStr=Inherit: Same as input
  Constant2=-1 : Constant  Value=-1
  Constant=-1 : Constant  Value=-1
  Data Inputs : Subsystem
  Demux : Demux  Outputs=7
  Integrator{,1..3} (4 alike) : Integrator
  Math Function : Math  Operator=pow  SaturateOnIntegerOverflow=on
  Math Function1 : Math  Operator=pow  SaturateOnIntegerOverflow=on
  Scope1 : Scope
      settings: SaveName=ScopeData4
  Sum : Sum  Inputs=|++  SaturateOnIntegerOverflow=on  InputSameDT=on  OutDataTypeStr=Inherit: Same as first input
  Sum2 : Sum  Inputs=|++++-+  SaturateOnIntegerOverflow=on  InputSameDT=on  OutDataTypeStr=Inherit: Same as first input
  Sum3 : Sum  Inputs=|+-  SaturateOnIntegerOverflow=on  InputSameDT=on  OutDataTypeStr=Inherit: Same as first input
  Sum4 : Sum  Inputs=|++---  SaturateOnIntegerOverflow=on  InputSameDT=on  OutDataTypeStr=Inherit: Same as first input
  Sum5 : Sum  Inputs=|+-  SaturateOnIntegerOverflow=on  InputSameDT=on  OutDataTypeStr=Inherit: Same as first input
  c0*(dz1-dz2) : Product  SaturateOnIntegerOverflow=on  RndMeth=Zero  InputSameDT=on  OutDataTypeStr=Inherit: Same as first input
  gain2=-1 : Gain  Gain=-1  SaturateOnIntegerOverflow=on  OutDataTypeStr=Inherit: Same as input  ParamDataTypeStr=Inherit: Same as input
  gain3=-1 : Gain  Gain=-1  SaturateOnIntegerOverflow=on  OutDataTypeStr=Inherit: Same as input  ParamDataTypeStr=Inherit: Same as input
  gain4=-1 : Gain  Gain=-1  SaturateOnIntegerOverflow=on  OutDataTypeStr=Inherit: Same as input  ParamDataTypeStr=Inherit: Same as input
  k1*(z1-q) : Product  SaturateOnIntegerOverflow=on  RndMeth=Zero  InputSameDT=on  OutDataTypeStr=Inherit: Same as first input
  k2*(z1-z2) : Product  SaturateOnIntegerOverflow=on  RndMeth=Zero  InputSameDT=on  OutDataTypeStr=Inherit: Same as first input
  m1ddz1/m1 : Product  SaturateOnIntegerOverflow=on  RndMeth=Zero  InputSameDT=on  OutDataTypeStr=Inherit: Same as first input
  m1g : Product  SaturateOnIntegerOverflow=on  RndMeth=Zero  InputSameDT=on  OutDataTypeStr=Inherit: Same as first input
  m2*ddz2/m2 : Product  SaturateOnIntegerOverflow=on  RndMeth=Zero  InputSameDT=on  OutDataTypeStr=Inherit: Same as first input
  m2g : Product  SaturateOnIntegerOverflow=on  RndMeth=Zero  InputSameDT=on  OutDataTypeStr=Inherit: Same as first input
  Out1 : Outport
  Out2 : Outport  Port=2
  Out3 : Outport  Port=3
  wires:
  Data Inputs/1("Simulaiton Parameters ") -> Demux/1
  Demux/1 -> m1g/1, Math Function/1
  Integrator2/1 -> Sum/2, Integrator/1
  Integrator/1 -> Sum5/1, Sum3/1
  siła amortyzatora/1 -> c0*(dz1-dz2)/2
  -1/1 -> Sum/1
  Sum/1 -> c0*(dz1-dz2)/1
  Integrator1/1 -> -1/1, Integrator3/1
  Demux/4 -> k2*(z1-z2)/2
  Demux/3 -> k1*(z1-q)/2
  Sum3/1 -> k1*(z1-q)/1, Out2/1
  Sum2/1 -> gain2=-1/1
  gain2=-1/1 -> m1ddz1/m1/2
  k1*(z1-q)/1 -> Sum2/1
  k2*(z1-z2)/1 -> Sum2/2, gain4=-1/1
  c0*(dz1-dz2)/1 -> Sum2/3, gain3=-1/1
  fd/1 -> Sum2/6, Sum4/3
  Constant=-1/1 -> Math Function/2
  Math Function/1 -> m1ddz1/m1/1
  m1ddz1/m1/1 -> Integrator2/1
  Demux/6 -> Sum2/4, Sum4/2
  gain3=-1/1 -> Sum4/5
  gain4=-1/1 -> Sum4/4
  Sum4/1 -> m2*ddz2/m2/1
  Demux/7 -> m1g/2, m2g/2
  Masa przypadająca na koło/1 -> m2g/1, Math Function1/1
  m1g/1 -> Sum2/5
  m2g/1 -> Sum4/1
  Constant2=-1/1 -> Math Function1/2
  Math Function1/1 -> m2*ddz2/m2/2, Scope1/1
  m2*ddz2/m2/1 -> Integrator1/1, Out1/1
  Integrator3/1 -> Sum5/2
  Sum5/1 -> k2*(z1-z2)/1, Out3/1
  q/1 -> Sum3/2

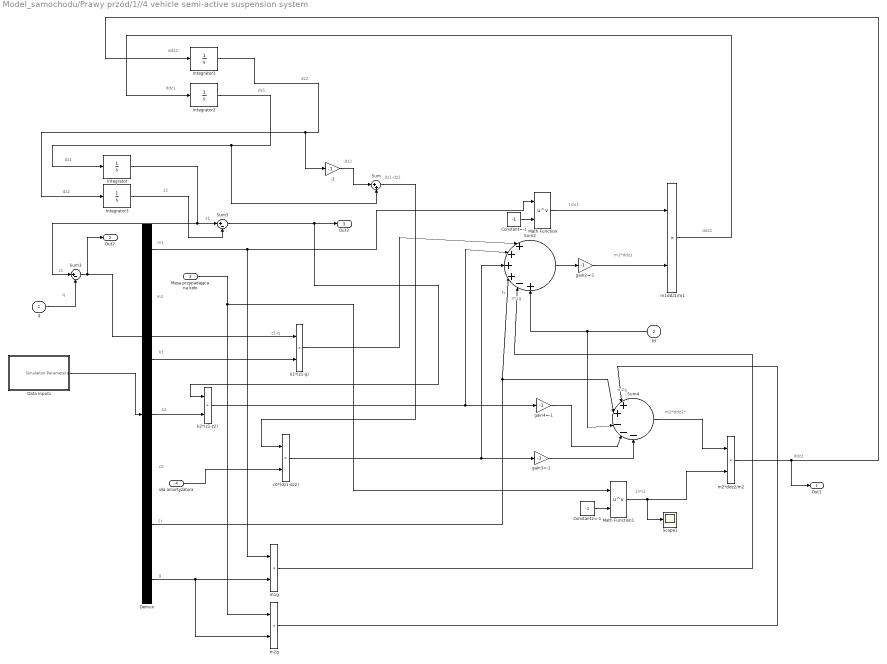
== system Model_samochodu/Prawy przód/1//4 vehicle semi-active suspension system ==
  note: m1
  note: k1
  note: m2
  note: k2
  note: c0
  note: z1
  note: dz1
  note: Fr
  note: g
  note: dz2
  note: -dz2
  note: dz1-dz2
  note: dz1
  note: dz2
  note: ddz2
  note: q
  note: z1
  note: z1-q
  note: Fr
  note: m1g
  note: m1*ddz1
  note: 1/m1
  note: ddz1
  note: m2g
  note: m2*ddz2*
  note: 1/m2
  note: ddz2
  note: z2
  note: ddz1
  q : Inport
  fd : Inport  Port=2
  Masa przypadająca na koło : Inport  Port=3
  siła amortyzatora : Inport  Port=4
  -1 : Gain  Gain=-1  SaturateOnIntegerOverflow=on  OutDataTypeStr=Inherit: Same as input  ParamDataTypeStr=Inherit: Same as input
  Constant2=-1 : Constant  Value=-1
  Constant=-1 : Constant  Value=-1
  Data Inputs : Subsystem
  Demux : Demux  Outputs=7
  Integrator{,1..3} (4 alike) : Integrator
  Math Function : Math  Operator=pow  SaturateOnIntegerOverflow=on
  Math Function1 : Math  Operator=pow  SaturateOnIntegerOverflow=on
  Scope1 : Scope
      settings: SaveName=ScopeData4
  Sum : Sum  Inputs=|++  SaturateOnIntegerOverflow=on  InputSameDT=on  OutDataTypeStr=Inherit: Same as first input
  Sum2 : Sum  Inputs=|++++-+  SaturateOnIntegerOverflow=on  InputSameDT=on  OutDataTypeStr=Inherit: Same as first input
  Sum3 : Sum  Inputs=|+-  SaturateOnIntegerOverflow=on  InputSameDT=on  OutDataTypeStr=Inherit: Same as first input
  Sum4 : Sum  Inputs=|++---  SaturateOnIntegerOverflow=on  InputSameDT=on  OutDataTypeStr=Inherit: Same as first input
  Sum5 : Sum  Inputs=|+-  SaturateOnIntegerOverflow=on  InputSameDT=on  OutDataTypeStr=Inherit: Same as first input
  c0*(dz1-dz2) : Product  SaturateOnIntegerOverflow=on  RndMeth=Zero  InputSameDT=on  OutDataTypeStr=Inherit: Same as first input
  gain2=-1 : Gain  Gain=-1  SaturateOnIntegerOverflow=on  OutDataTypeStr=Inherit: Same as input  ParamDataTypeStr=Inherit: Same as input
  gain3=-1 : Gain  Gain=-1  SaturateOnIntegerOverflow=on  OutDataTypeStr=Inherit: Same as input  ParamDataTypeStr=Inherit: Same as input
  gain4=-1 : Gain  Gain=-1  SaturateOnIntegerOverflow=on  OutDataTypeStr=Inherit: Same as input  ParamDataTypeStr=Inherit: Same as input
  k1*(z1-q) : Product  SaturateOnIntegerOverflow=on  RndMeth=Zero  InputSameDT=on  OutDataTypeStr=Inherit: Same as first input
  k2*(z1-z2) : Product  SaturateOnIntegerOverflow=on  RndMeth=Zero  InputSameDT=on  OutDataTypeStr=Inherit: Same as first input
  m1ddz1/m1 : Product  SaturateOnIntegerOverflow=on  RndMeth=Zero  InputSameDT=on  OutDataTypeStr=Inherit: Same as first input
  m1g : Product  SaturateOnIntegerOverflow=on  RndMeth=Zero  InputSameDT=on  OutDataTypeStr=Inherit: Same as first input
  m2*ddz2/m2 : Product  SaturateOnIntegerOverflow=on  RndMeth=Zero  InputSameDT=on  OutDataTypeStr=Inherit: Same as first input
  m2g : Product  SaturateOnIntegerOverflow=on  RndMeth=Zero  InputSameDT=on  OutDataTypeStr=Inherit: Same as first input
  Out1 : Outport
  Out2 : Outport  Port=2
  Out3 : Outport  Port=3
  wires:
  Data Inputs/1("Simulaiton Parameters ") -> Demux/1
  Demux/1 -> m1g/1, Math Function/1
  Integrator2/1 -> Sum/2, Integrator/1
  Integrator/1 -> Sum5/1, Sum3/1
  siła amortyzatora/1 -> c0*(dz1-dz2)/2
  -1/1 -> Sum/1
  Sum/1 -> c0*(dz1-dz2)/1
  Integrator1/1 -> -1/1, Integrator3/1
  Demux/4 -> k2*(z1-z2)/2
  Demux/3 -> k1*(z1-q)/2
  Sum3/1 -> k1*(z1-q)/1, Out2/1
  Sum2/1 -> gain2=-1/1
  gain2=-1/1 -> m1ddz1/m1/2
  k1*(z1-q)/1 -> Sum2/1
  k2*(z1-z2)/1 -> Sum2/2, gain4=-1/1
  c0*(dz1-dz2)/1 -> Sum2/3, gain3=-1/1
  fd/1 -> Sum2/6, Sum4/3
  Constant=-1/1 -> Math Function/2
  Math Function/1 -> m1ddz1/m1/1
  m1ddz1/m1/1 -> Integrator2/1
  Demux/6 -> Sum2/4, Sum4/2
  gain3=-1/1 -> Sum4/5
  gain4=-1/1 -> Sum4/4
  Sum4/1 -> m2*ddz2/m2/1
  Demux/7 -> m1g/2, m2g/2
  Masa przypadająca na koło/1 -> m2g/1, Math Function1/1
  m1g/1 -> Sum2/5
  m2g/1 -> Sum4/1
  Constant2=-1/1 -> Math Function1/2
  Math Function1/1 -> m2*ddz2/m2/2, Scope1/1
  m2*ddz2/m2/1 -> Integrator1/1, Out1/1
  Integrator3/1 -> Sum5/2
  Sum5/1 -> k2*(z1-z2)/1, Out3/1
  q/1 -> Sum3/2

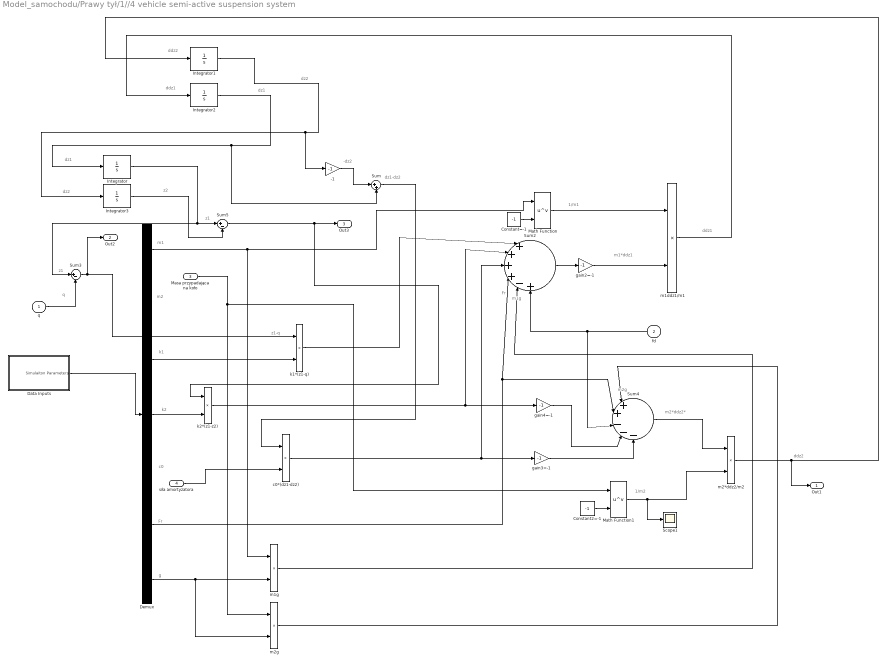
== system Model_samochodu/Prawy tył/1//4 vehicle semi-active suspension system ==
  note: m1
  note: k1
  note: m2
  note: k2
  note: c0
  note: z1
  note: dz1
  note: Fr
  note: g
  note: dz2
  note: -dz2
  note: dz1-dz2
  note: dz1
  note: dz2
  note: ddz2
  note: q
  note: z1
  note: z1-q
  note: Fr
  note: m1g
  note: m1*ddz1
  note: 1/m1
  note: ddz1
  note: m2g
  note: m2*ddz2*
  note: 1/m2
  note: ddz2
  note: z2
  note: ddz1
  q : Inport
  fd : Inport  Port=2
  Masa przypadająca na koło : Inport  Port=3
  siła amortyzatora : Inport  Port=4
  -1 : Gain  Gain=-1  SaturateOnIntegerOverflow=on  OutDataTypeStr=Inherit: Same as input  ParamDataTypeStr=Inherit: Same as input
  Constant2=-1 : Constant  Value=-1
  Constant=-1 : Constant  Value=-1
  Data Inputs : Subsystem
  Demux : Demux  Outputs=7
  Integrator{,1..3} (4 alike) : Integrator
  Math Function : Math  Operator=pow  SaturateOnIntegerOverflow=on
  Math Function1 : Math  Operator=pow  SaturateOnIntegerOverflow=on
  Scope1 : Scope
      settings: SaveName=ScopeData4
  Sum : Sum  Inputs=|++  SaturateOnIntegerOverflow=on  InputSameDT=on  OutDataTypeStr=Inherit: Same as first input
  Sum2 : Sum  Inputs=|++++-+  SaturateOnIntegerOverflow=on  InputSameDT=on  OutDataTypeStr=Inherit: Same as first input
  Sum3 : Sum  Inputs=|+-  SaturateOnIntegerOverflow=on  InputSameDT=on  OutDataTypeStr=Inherit: Same as first input
  Sum4 : Sum  Inputs=|++---  SaturateOnIntegerOverflow=on  InputSameDT=on  OutDataTypeStr=Inherit: Same as first input
  Sum5 : Sum  Inputs=|+-  SaturateOnIntegerOverflow=on  InputSameDT=on  OutDataTypeStr=Inherit: Same as first input
  c0*(dz1-dz2) : Product  SaturateOnIntegerOverflow=on  RndMeth=Zero  InputSameDT=on  OutDataTypeStr=Inherit: Same as first input
  gain2=-1 : Gain  Gain=-1  SaturateOnIntegerOverflow=on  OutDataTypeStr=Inherit: Same as input  ParamDataTypeStr=Inherit: Same as input
  gain3=-1 : Gain  Gain=-1  SaturateOnIntegerOverflow=on  OutDataTypeStr=Inherit: Same as input  ParamDataTypeStr=Inherit: Same as input
  gain4=-1 : Gain  Gain=-1  SaturateOnIntegerOverflow=on  OutDataTypeStr=Inherit: Same as input  ParamDataTypeStr=Inherit: Same as input
  k1*(z1-q) : Product  SaturateOnIntegerOverflow=on  RndMeth=Zero  InputSameDT=on  OutDataTypeStr=Inherit: Same as first input
  k2*(z1-z2) : Product  SaturateOnIntegerOverflow=on  RndMeth=Zero  InputSameDT=on  OutDataTypeStr=Inherit: Same as first input
  m1ddz1/m1 : Product  SaturateOnIntegerOverflow=on  RndMeth=Zero  InputSameDT=on  OutDataTypeStr=Inherit: Same as first input
  m1g : Product  SaturateOnIntegerOverflow=on  RndMeth=Zero  InputSameDT=on  OutDataTypeStr=Inherit: Same as first input
  m2*ddz2/m2 : Product  SaturateOnIntegerOverflow=on  RndMeth=Zero  InputSameDT=on  OutDataTypeStr=Inherit: Same as first input
  m2g : Product  SaturateOnIntegerOverflow=on  RndMeth=Zero  InputSameDT=on  OutDataTypeStr=Inherit: Same as first input
  Out1 : Outport
  Out2 : Outport  Port=2
  Out3 : Outport  Port=3
  wires:
  Data Inputs/1("Simulaiton Parameters ") -> Demux/1
  Demux/1 -> m1g/1, Math Function/1
  Integrator2/1 -> Sum/2, Integrator/1
  Integrator/1 -> Sum5/1, Sum3/1
  siła amortyzatora/1 -> c0*(dz1-dz2)/2
  -1/1 -> Sum/1
  Sum/1 -> c0*(dz1-dz2)/1
  Integrator1/1 -> -1/1, Integrator3/1
  Demux/4 -> k2*(z1-z2)/2
  Demux/3 -> k1*(z1-q)/2
  Sum3/1 -> k1*(z1-q)/1, Out2/1
  Sum2/1 -> gain2=-1/1
  gain2=-1/1 -> m1ddz1/m1/2
  k1*(z1-q)/1 -> Sum2/1
  k2*(z1-z2)/1 -> Sum2/2, gain4=-1/1
  c0*(dz1-dz2)/1 -> Sum2/3, gain3=-1/1
  fd/1 -> Sum2/6, Sum4/3
  Constant=-1/1 -> Math Function/2
  Math Function/1 -> m1ddz1/m1/1
  m1ddz1/m1/1 -> Integrator2/1
  Demux/6 -> Sum2/4, Sum4/2
  gain3=-1/1 -> Sum4/5
  gain4=-1/1 -> Sum4/4
  Sum4/1 -> m2*ddz2/m2/1
  Demux/7 -> m1g/2, m2g/2
  Masa przypadająca na koło/1 -> m2g/1, Math Function1/1
  m1g/1 -> Sum2/5
  m2g/1 -> Sum4/1
  Constant2=-1/1 -> Math Function1/2
  Math Function1/1 -> m2*ddz2/m2/2, Scope1/1
  m2*ddz2/m2/1 -> Integrator1/1, Out1/1
  Integrator3/1 -> Sum5/2
  Sum5/1 -> k2*(z1-z2)/1, Out3/1
  q/1 -> Sum3/2

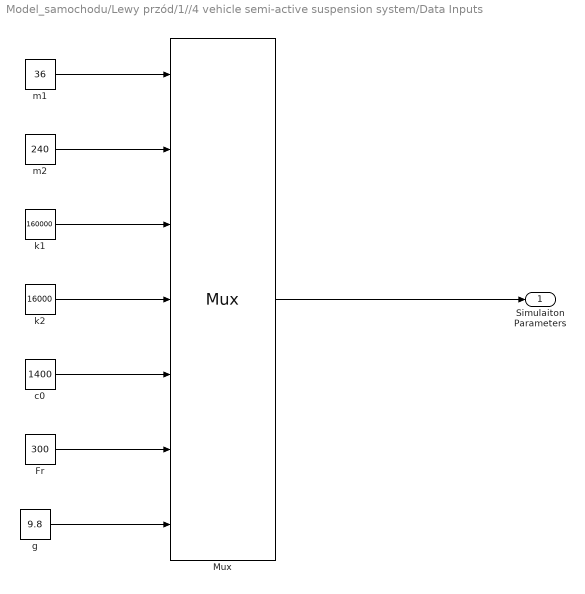
== system Model_samochodu/Lewy przód/1//4 vehicle semi-active suspension system/Data Inputs ==
  Fr : Constant  Value=300
  Mux : Mux  Inputs=7
  c0 : Constant  Value=1400
  g : Constant  Value=9.8
  k1 : Constant  Value=160000
  k2 : Constant  Value=16000
  m1 : Constant  Value=36
  m2 : Constant  Value=240
  "Simulaiton Parameters " : Outport
  wires:
  m1/1 -> Mux/1
  m2/1 -> Mux/2
  k1/1 -> Mux/3
  k2/1 -> Mux/4
  c0/1 -> Mux/5
  Fr/1 -> Mux/6
  g/1 -> Mux/7
  Mux/1 -> "Simulaiton Parameters "/1

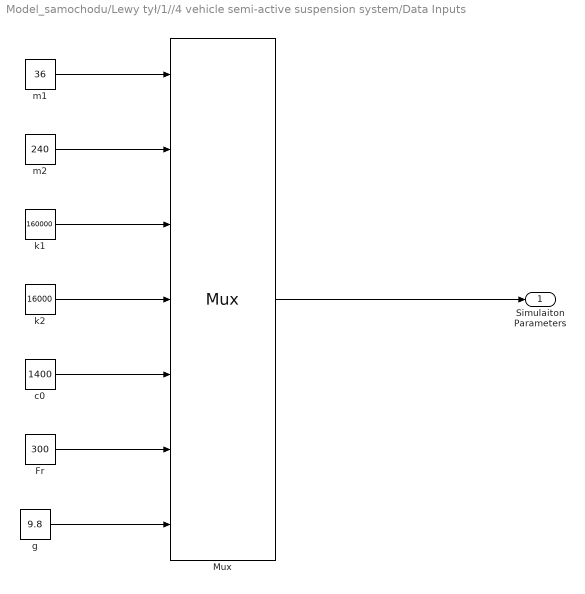
== system Model_samochodu/Lewy tył/1//4 vehicle semi-active suspension system/Data Inputs ==
  Fr : Constant  Value=300
  Mux : Mux  Inputs=7
  c0 : Constant  Value=1400
  g : Constant  Value=9.8
  k1 : Constant  Value=160000
  k2 : Constant  Value=16000
  m1 : Constant  Value=36
  m2 : Constant  Value=240
  "Simulaiton Parameters " : Outport
  wires:
  m1/1 -> Mux/1
  m2/1 -> Mux/2
  k1/1 -> Mux/3
  k2/1 -> Mux/4
  c0/1 -> Mux/5
  Fr/1 -> Mux/6
  g/1 -> Mux/7
  Mux/1 -> "Simulaiton Parameters "/1

== system Model_samochodu/Prawy przód/1//4 vehicle semi-active suspension system/Data Inputs ==
  Fr : Constant  Value=300
  Mux : Mux  Inputs=7
  c0 : Constant  Value=1400
  g : Constant  Value=9.8
  k1 : Constant  Value=160000
  k2 : Constant  Value=16000
  m1 : Constant  Value=36
  m2 : Constant  Value=240
  "Simulaiton Parameters " : Outport
  wires:
  m1/1 -> Mux/1
  m2/1 -> Mux/2
  k1/1 -> Mux/3
  k2/1 -> Mux/4
  c0/1 -> Mux/5
  Fr/1 -> Mux/6
  g/1 -> Mux/7
  Mux/1 -> "Simulaiton Parameters "/1

== system Model_samochodu/Prawy tył/1//4 vehicle semi-active suspension system/Data Inputs ==
  Fr : Constant  Value=300
  Mux : Mux  Inputs=7
  c0 : Constant  Value=1400
  g : Constant  Value=9.8
  k1 : Constant  Value=160000
  k2 : Constant  Value=16000
  m1 : Constant  Value=36
  m2 : Constant  Value=240
  "Simulaiton Parameters " : Outport
  wires:
  m1/1 -> Mux/1
  m2/1 -> Mux/2
  k1/1 -> Mux/3
  k2/1 -> Mux/4
  c0/1 -> Mux/5
  Fr/1 -> Mux/6
  g/1 -> Mux/7
  Mux/1 -> "Simulaiton Parameters "/1
